simulink model "testTorqueFree"  (R2021a)
settings: Solver=VariableStepAuto  StartTime=0.0  StopTime=Torb  RelTol=1e-3
libraries: sharedtransform x1
settings Model: DataDictionary=databus.sldd  Creator=Laura  LastModifiedBy=Laura

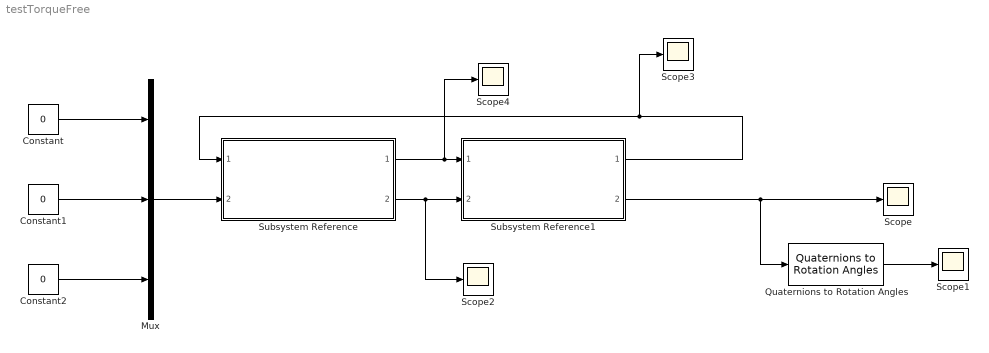
== system testTorqueFree ==
  Constant : Constant  Value=0
  Constant1 : Constant  Value=0
  Constant2 : Constant  Value=0
  Mux : Mux  Inputs=3
  Quaternions to Rotation Angles : sharedtransform/Quaternions to Rotation Angles  rotationOrder=ZYX  aMode=aMode
      settings: SourceProductBaseCode=AE,PW,DR,MT,UV,VE
  Scope{,1..4} (5 alike) : Scope
  Subsystem Reference : Subsystem  ReferencedSubsystem=Dynamics
  Subsystem Reference1 : Subsystem  ReferencedSubsystem=Kinematics
  wires:
  Quaternions to Rotation Angles/1 -> Scope1/1
  Mux/1 -> Subsystem Reference/2
  Subsystem Reference1/1 -> Scope3/1, Subsystem Reference/1
  Subsystem Reference1/2 -> Quaternions to Rotation Angles/1, Scope/1
  Subsystem Reference/2 -> Scope2/1, Subsystem Reference1/2
  Constant1/1 -> Mux/2
  Subsystem Reference/1 -> Scope4/1, Subsystem Reference1/1
  Constant2/1 -> Mux/3
  Constant/1 -> Mux/1
